simulink model "slidingSimulation"  (R2024a)
settings: Solver=ode4  StartTime=0.0  StopTime=10  FixedStep=1E-4  RelTol=1e-3
undefined symbols (not defined in the file or in its folder): initial_1, observer, sliding
settings Model: Creator=b_ant  LastModifiedBy=b_ant

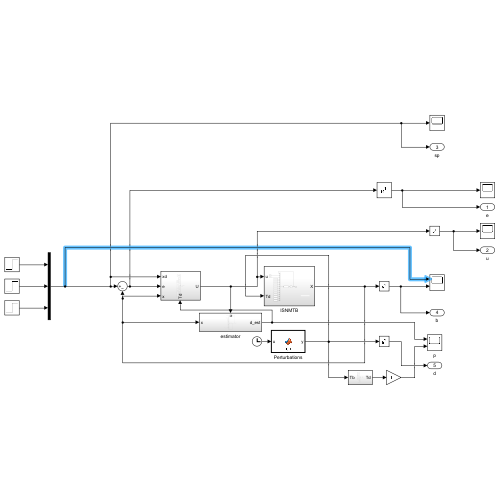
[thumbnail: Simulink's stored preview of the top-level diagram]
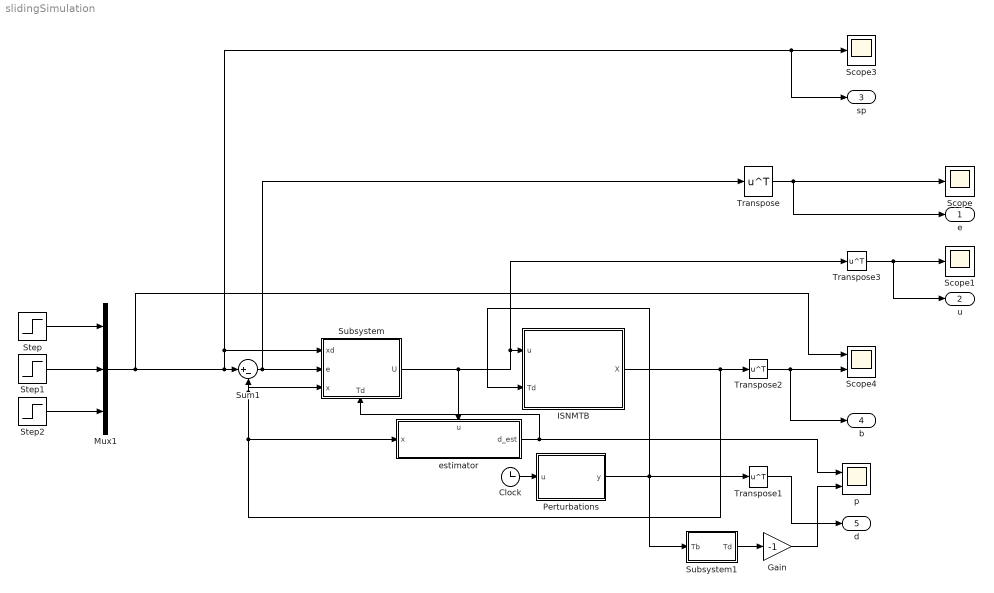
== system slidingSimulation ==
  Clock : Clock
      settings: Decimation=1000
  Gain : Gain  Gain=-1
  ISNMTB : Subsystem
  Mux1 : Mux  Inputs=3
  Perturbations : MATLAB Function  TreatAsAtomicUnit=on
  Scope : Scope
  Scope1 : Scope
  Scope3 : Scope
  Scope4 : Scope  NumInputPorts=2
  Step : Step  Time=0.01  SampleTime=0
  Step1 : Step  Time=0.01  SampleTime=0
  Step2 : Step  Time=0.01  SampleTime=0
  Subsystem : Subsystem
      settings: PortSchema="{\"entries\":[{\"content\":{\"sides\":[{\"content\":{\"connectorIds\":[\"In1\",\"In2\",\"In3\"]},\"type\":\"ConnectorPlacement.EquallySpacedRectSide\",\"uuid\":\"8dd7d522-9b9c-45d9-b832-502a96d333e6\"},{\"content\":{\"connectorIds\":[\"Out1\"],\"side\":\"RIGHT\"},\"type\":\"ConnectorPlacement.EquallySpacedRectSide\",\"uuid\":\"030ab568-8b67-42ae-ab9d-0e2e0fb94543\"},{\"content\":{\"side\":\"TOP\"},\"type\":\"ConnectorPlacement.EquallySpacedRectSide\",\"uuid\":\"4f617b28-94a1-4a3d-8f94-23e58ede5e34\"},{\"content\":{\"connectorIds\":[\"In4\"],\"side\":\"BOTTOM\"},\"type\":\"ConnectorPlacement.EquallySpacedRectSide\",\"uuid\":\"1fe40258-6e88-4733-8d2c-f23cf23aef95\"}]},\"type\":\"ConnectorPlacement.EquallySpacedConnector\",\"uuid\":\"c1f31e5d-b9fa-4e41-a0e3-4e1d75fca667\"}],\"packageUris\":[\"http://schema.mathworks.com/mf0/Connector/R2020b\"],\"version\":\"1.0\"}"
  Subsystem1 : Subsystem
  Sum1 : Sum  Inputs=|+-
  Transpose{,1..3} (4 alike) : Math  Operator=transpose
  estimator : Subsystem
      settings: PortSchema="{\"entries\":[{\"content\":{\"sides\":[{\"content\":{\"connectorIds\":[\"In1\"]},\"type\":\"ConnectorPlacement.EquallySpacedRectSide\",\"uuid\":\"f9e844d6-ee13-4ae8-8d73-084dc6b9c230\"},{\"content\":{\"connectorIds\":[\"Out1\"],\"side\":\"RIGHT\"},\"type\":\"ConnectorPlacement.EquallySpacedRectSide\",\"uuid\":\"c081e574-2129-4344-8b67-56cd55c23b50\"},{\"content\":{\"connectorIds\":[\"In2\"],\"side\":\"TOP\"},\"type\":\"ConnectorPlacement.EquallySpacedRectSide\",\"uuid\":\"bf6f2985-e51e-41d0-a8b1-b5505659e5f3\"},{\"content\":{\"side\":\"BOTTOM\"},\"type\":\"ConnectorPlacement.EquallySpacedRectSide\",\"uuid\":\"e1697b77-960b-449d-843b-5909cf972339\"}]},\"type\":\"ConnectorPlacement.EquallySpacedConnector\",\"uuid\":\"c9da1c41-5311-41bf-ab5b-06506202d90f\"}],\"packageUris\":[\"http://schema.mathworks.com/mf0/Connector/R2020b\"],\"version\":\"1.0\"}"
  p : Scope  NumInputPorts=2
  e : Outport
  u : Outport  Port=2
  sp : Outport  Port=3
  b : Outport  Port=4
  d : Outport  Port=5
  wires:
  Transpose/1 -> e/1, Scope/1
  Step/1 -> Mux1/1
  Step1/1 -> Mux1/2
  Transpose2/1 -> b/1, Scope4/2
  Transpose3/1 -> u/1, Scope1/1
  ISNMTB/1(X) -> estimator/1(x), Subsystem/3(x), Sum1/2, Transpose2/1
  Clock/1 -> Perturbations/1(u)
  Transpose1/1 -> d/1
  Step2/1 -> Mux1/3
  Sum1/1 -> Transpose/1, Subsystem/2(e)
  Mux1/1 -> sp/1, Scope3/1, Subsystem/1(xd), Sum1/1, Scope4/1
  Perturbations/1(y) -> ISNMTB/2(Td), Transpose1/1, Subsystem1/1(Tb)
  estimator/1(d_est) -> p/1, Subsystem/4(Td)
  Subsystem/1(U) -> Transpose3/1, ISNMTB/1(u), estimator/2(u)
  Subsystem1/1(Td) -> Gain/1
  Gain/1 -> p/2

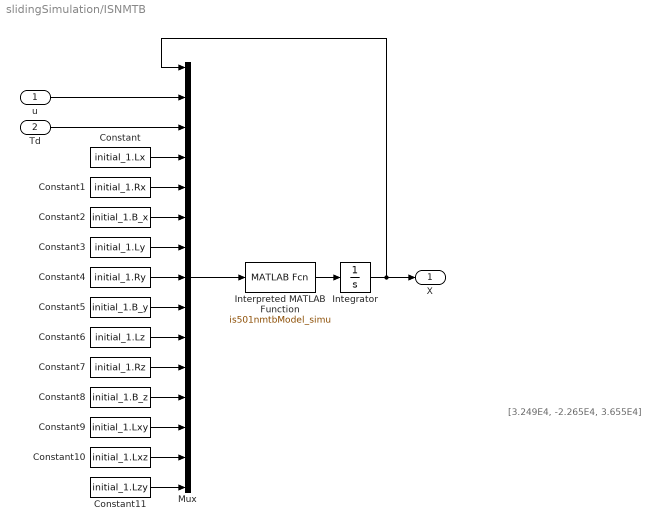
== system slidingSimulation/ISNMTB ==
  note: [3.249E4, -2.265E4, 3.655E4]
  u : Inport
  Td : Inport  Port=2
  Constant : Constant  Value=initial_1.Lx
  Constant1 : Constant  Value=initial_1.Rx
  Constant10 : Constant  Value=initial_1.Lxz
  Constant11 : Constant  Value=initial_1.Lzy
  Constant2 : Constant  Value=initial_1.B_x
  Constant3 : Constant  Value=initial_1.Ly
  Constant4 : Constant  Value=initial_1.Ry
  Constant5 : Constant  Value=initial_1.B_y
  Constant6 : Constant  Value=initial_1.Lz
  Constant7 : Constant  Value=initial_1.Rz
  Constant8 : Constant  Value=initial_1.B_z
  Constant9 : Constant  Value=initial_1.Lxy
  Integrator : Integrator  InitialCondition=[3.249E4, -2.265E4, 3.655E4]
  Interpreted MATLAB Function : MATLABFcn  MATLABFcn=is501nmtbModel_simu  OutputDimensions=3
  Mux : Mux  Inputs=15
  X : Outport
  wires:
  Interpreted MATLAB Function/1 -> Integrator/1
  Integrator/1 -> X/1, Mux/1
  Mux/1 -> Interpreted MATLAB Function/1
  u/1 -> Mux/2
  Td/1 -> Mux/3
  Constant/1 -> Mux/4
  Constant1/1 -> Mux/5
  Constant2/1 -> Mux/6
  Constant3/1 -> Mux/7
  Constant4/1 -> Mux/8
  Constant5/1 -> Mux/9
  Constant6/1 -> Mux/10
  Constant7/1 -> Mux/11
  Constant8/1 -> Mux/12
  Constant9/1 -> Mux/13
  Constant10/1 -> Mux/14
  Constant11/1 -> Mux/15

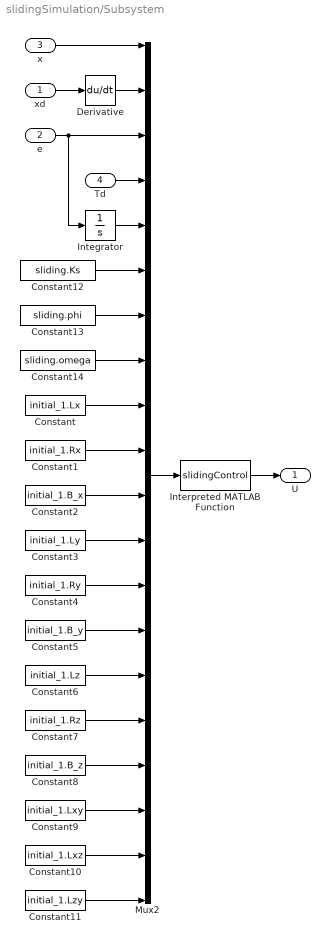
== system slidingSimulation/Subsystem ==
  xd : Inport
  e : Inport  Port=2
  x : Inport  Port=3
  Td : Inport  Port=4
  Constant : Constant  Value=initial_1.Lx
  Constant1 : Constant  Value=initial_1.Rx
  Constant10 : Constant  Value=initial_1.Lxz
  Constant11 : Constant  Value=initial_1.Lzy
  Constant12 : Constant  Value=sliding.Ks
  Constant13 : Constant  Value=sliding.phi
  Constant14 : Constant  Value=sliding.omega
  Constant2 : Constant  Value=initial_1.B_x
  Constant3 : Constant  Value=initial_1.Ly
  Constant4 : Constant  Value=initial_1.Ry
  Constant5 : Constant  Value=initial_1.B_y
  Constant6 : Constant  Value=initial_1.Lz
  Constant7 : Constant  Value=initial_1.Rz
  Constant8 : Constant  Value=initial_1.B_z
  Constant9 : Constant  Value=initial_1.Lxy
  Derivative : Derivative
  Integrator : Integrator
  Interpreted MATLAB Function : MATLABFcn  MATLABFcn=slidingControl  OutputDimensions=3
  Mux2 : Mux  Inputs=20
  U : Outport
  wires:
  Interpreted MATLAB Function/1 -> U/1
  x/1 -> Mux2/1
  Derivative/1 -> Mux2/2
  e/1 -> Mux2/3, Integrator/1
  Td/1 -> Mux2/4
  Constant11/1 -> Mux2/20
  Constant10/1 -> Mux2/19
  Constant9/1 -> Mux2/18
  Constant8/1 -> Mux2/17
  Constant7/1 -> Mux2/16
  Constant6/1 -> Mux2/15
  Constant5/1 -> Mux2/14
  Constant4/1 -> Mux2/13
  Constant3/1 -> Mux2/12
  Constant2/1 -> Mux2/11
  Constant1/1 -> Mux2/10
  Constant/1 -> Mux2/9
  xd/1 -> Derivative/1
  Integrator/1 -> Mux2/5
  Constant12/1 -> Mux2/6
  Constant13/1 -> Mux2/7
  Constant14/1 -> Mux2/8
  Mux2/1 -> Interpreted MATLAB Function/1

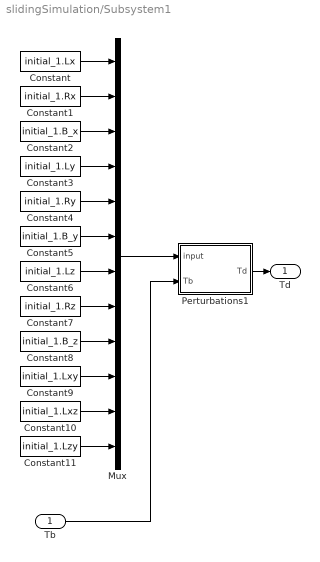
== system slidingSimulation/Subsystem1 ==
  Tb : Inport
  Constant : Constant  Value=initial_1.Lx
  Constant1 : Constant  Value=initial_1.Rx
  Constant10 : Constant  Value=initial_1.Lxz
  Constant11 : Constant  Value=initial_1.Lzy
  Constant2 : Constant  Value=initial_1.B_x
  Constant3 : Constant  Value=initial_1.Ly
  Constant4 : Constant  Value=initial_1.Ry
  Constant5 : Constant  Value=initial_1.B_y
  Constant6 : Constant  Value=initial_1.Lz
  Constant7 : Constant  Value=initial_1.Rz
  Constant8 : Constant  Value=initial_1.B_z
  Constant9 : Constant  Value=initial_1.Lxy
  Mux : Mux  Inputs=12
  Perturbations1 : MATLAB Function  TreatAsAtomicUnit=on
  Td : Outport
  wires:
  Constant2/1 -> Mux/3
  Constant6/1 -> Mux/7
  Constant7/1 -> Mux/8
  Constant8/1 -> Mux/9
  Constant9/1 -> Mux/10
  Constant/1 -> Mux/1
  Constant11/1 -> Mux/12
  Constant10/1 -> Mux/11
  Constant5/1 -> Mux/6
  Constant3/1 -> Mux/4
  Mux/1 -> Perturbations1/1(input)
  Constant1/1 -> Mux/2
  Constant4/1 -> Mux/5
  Tb/1 -> Perturbations1/2(Tb)
  Perturbations1/1(Td) -> Td/1

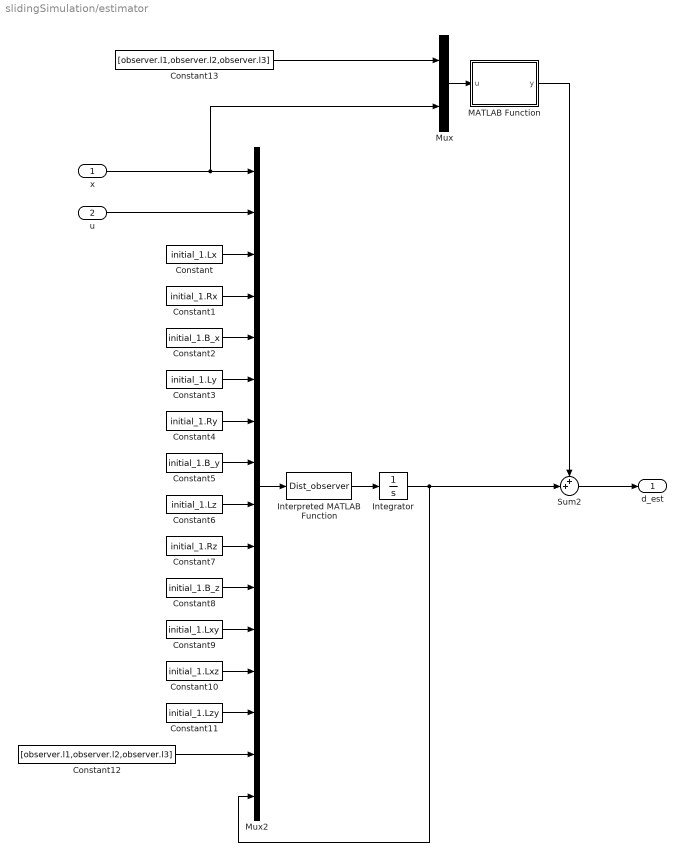
== system slidingSimulation/estimator ==
  x : Inport
  u : Inport  Port=2
  Constant : Constant  Value=initial_1.Lx
  Constant1 : Constant  Value=initial_1.Rx
  Constant10 : Constant  Value=initial_1.Lxz
  Constant11 : Constant  Value=initial_1.Lzy
  Constant12 : Constant  Value=[observer.l1,observer.l2,observer.l3]
  Constant13 : Constant  Value=[observer.l1,observer.l2,observer.l3]
  Constant2 : Constant  Value=initial_1.B_x
  Constant3 : Constant  Value=initial_1.Ly
  Constant4 : Constant  Value=initial_1.Ry
  Constant5 : Constant  Value=initial_1.B_y
  Constant6 : Constant  Value=initial_1.Lz
  Constant7 : Constant  Value=initial_1.Rz
  Constant8 : Constant  Value=initial_1.B_z
  Constant9 : Constant  Value=initial_1.Lxy
  Integrator : Integrator  InitialCondition=[0,0,0]
  Interpreted MATLAB Function : MATLABFcn  MATLABFcn=Dist_observer  OutputDimensions=3
  MATLAB Function : MATLAB Function  TreatAsAtomicUnit=on
  Mux : Mux  Inputs=2
  Mux2 : Mux  Inputs=16
  Sum2 : Sum  Inputs=++|
  d_est : Outport
  wires:
  Constant6/1 -> Mux2/9
  MATLAB Function/1(y) -> Sum2/1
  Constant10/1 -> Mux2/13
  Integrator/1 -> Sum2/2, Mux2/16
  Interpreted MATLAB Function/1 -> Integrator/1
  Constant2/1 -> Mux2/5
  Constant4/1 -> Mux2/7
  Constant7/1 -> Mux2/10
  Mux2/1 -> Interpreted MATLAB Function/1
  Constant11/1 -> Mux2/14
  Constant8/1 -> Mux2/11
  Constant1/1 -> Mux2/4
  Constant3/1 -> Mux2/6
  Constant/1 -> Mux2/3
  Constant9/1 -> Mux2/12
  Constant5/1 -> Mux2/8
  Constant12/1 -> Mux2/15
  u/1 -> Mux2/2
  Sum2/1 -> d_est/1
  Constant13/1 -> Mux/1
  Mux/1 -> MATLAB Function/1(u)
  x/1 -> Mux/2, Mux2/1

== matlab function slidingSimulation/Perturbations ==
  data: u input; y output
function y = fcn(u)
y= [2.522*sin(2*pi*4.788E-3*u)+3.249E04;
   -5.174*sin(2*pi*7.481E-3*u)-2.265E04;
    3.359*sin(2*pi*8.378E-3*u)+3.655E04];
end

== matlab function slidingSimulation/Subsystem1/Perturbations1 ==
  data: input input; Td output; Tb input
function Td = fcn(input, Tb)
    Lxx =  input(1);
    Rx  =  input(2);
    B_1 =  input(3);
    Lyy =  input(4);
    Ry  =  input(5);
    B_2 =  input(6);
    Lzz =  input(7);
    Rz  =  input(8);
    B_3 =  input(9);
    Lxy =  input(10);
    Lxz =  input(11);
    Lzy =  input(12);

    %%%Parameter reading
    L1 =[Lxx, (B_1/B_2)*Lxy, (B_1/B_3)*Lxz;
        (B_2/B_1)*Lxy, Lyy, (B_2/B_3)*Lzy;
        (B_3/B_1)*Lxz, (B_3/B_2)*Lzy, Lzz];
    L = [Lxx, Lxy, Lxz;
         Lxy, Lyy, Lzy;
         Lxz, Lzy, Lzz];
    R = diag([Rx,Ry,Rz]);
    B = diag([B_1,B_2,B_3]);
    
    %%% Model matrix
    Ap = -inv(L1)*R;
    Bp =  B*inv(L)*1E9; 
    Td = Ap*Tb;
end

== matlab function slidingSimulation/estimator/MATLAB Function ==
  data: u input; y output
function y = fcn(u)
l = diag([u(1),u(2),u(3)]);
x = [u(4);u(5);u(6)];

y = l*x;
end
